simulink model "UWV_SIM"  (R2017a)
settings: Solver=FixedStepAuto  StartTime=0.0  StopTime=5  FixedStep=0.01  RelTol=1e-3  EnableMultiTasking=on
settings Model: Creator=Think  LastModifiedBy=Think
settings DataIOCC: LimitDataPoints=on  SaveFormat=Array
settings OptimizationCC: LifeSpan=inf
settings DebuggingCC: SolverPrmCheckMsg=warning  SFUnexpectedBacktrackingDiag=warning  SFNoUnconditionalDefaultTransitionDiag=warning  SFExecutionAtInitializationDiag=none
settings HardwareCC: ProdBitPerPointer=32  ProdBitPerSizeT=32  ProdBitPerPtrDiffT=32  ProdLargestAtomicFloat=None  ProdIntDivRoundTo=Undefined  ProdEndianess=Unspecified  ProdWordSize=32  ProdHWDeviceType=32-bit Generic
settings ModelReferenceCC: PropagateSignalLabelsOutOfModel=off
settings GRTTargetCC: TargetLangStandard=C89/C90 (ANSI)  GeneratePreprocessorConditionals=Disable all
settings ConfigComp: CovMetricSettings=dw  CovHtmlReporting=on  CovSaveCumulativeToWorkspaceVar=on  CovSaveSingleToWorkspaceVar=on  CovExternalEMLEnable=off  CovSFcnEnable=off

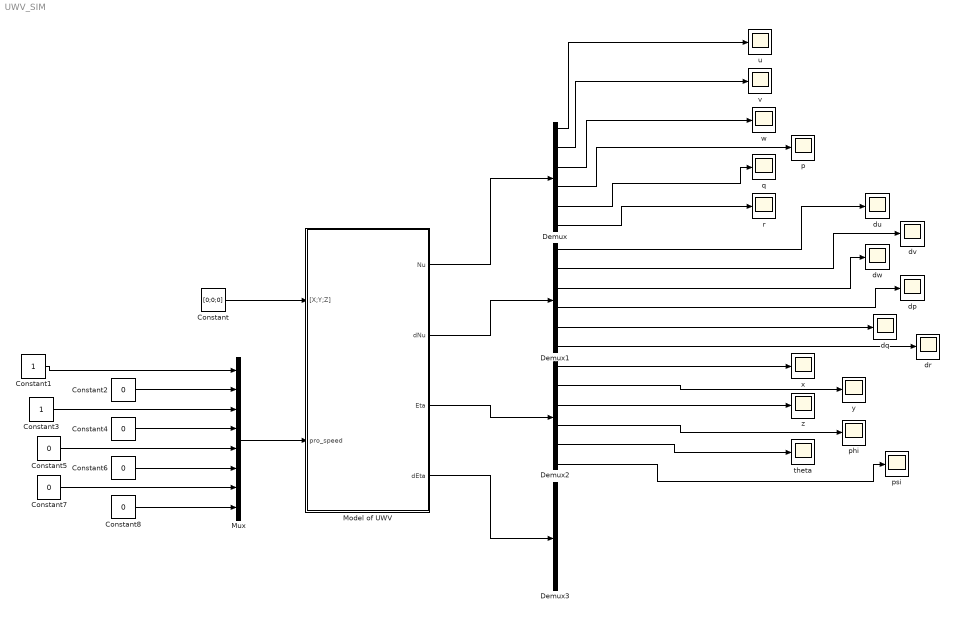
== system UWV_SIM ==
  Constant : Constant  Value=[0;0;0]
  Constant1 : Constant
  Constant{2,4..8} (6 alike) : Constant  Value=0
  Constant3 : Constant
  Demux{,1..3} (4 alike) : Demux  Outputs=6
  Model of UWV : Subsystem
  Mux : Mux  Inputs=8
  dp : Scope
  dq : Scope
  dr : Scope
  du : Scope
  dv : Scope
  dw : Scope
  p : Scope
  phi : Scope
  psi : Scope
  q : Scope
  r : Scope
  theta : Scope
  u : Scope
  v : Scope
  w : Scope
  x : Scope
  y : Scope
  z : Scope
  wires:
  Constant/1 -> Model of UWV/1("[X;Y;Z]")
  Mux/1 -> Model of UWV/2(pro_speed)
  Model of UWV/1(Nu) -> Demux/1
  Model of UWV/2(dNu) -> Demux1/1
  Model of UWV/3(Eta) -> Demux2/1
  Model of UWV/4(dEta) -> Demux3/1
  Demux/1 -> u/1
  Demux/2 -> v/1
  Demux/3 -> w/1
  Demux/4 -> p/1
  Demux/5 -> q/1
  Demux/6 -> r/1
  Demux1/1 -> du/1
  Demux1/2 -> dv/1
  Demux1/3 -> dw/1
  Demux1/4 -> dp/1
  Demux1/5 -> dq/1
  Demux1/6 -> dr/1
  Demux2/1 -> x/1
  Demux2/2 -> y/1
  Demux2/3 -> z/1
  Demux2/4 -> phi/1
  Demux2/5 -> theta/1
  Demux2/6 -> psi/1
  Constant1/1 -> Mux/1
  Constant3/1 -> Mux/3
  Constant5/1 -> Mux/5
  Constant7/1 -> Mux/7
  Constant2/1 -> Mux/2
  Constant4/1 -> Mux/4
  Constant6/1 -> Mux/6
  Constant8/1 -> Mux/8

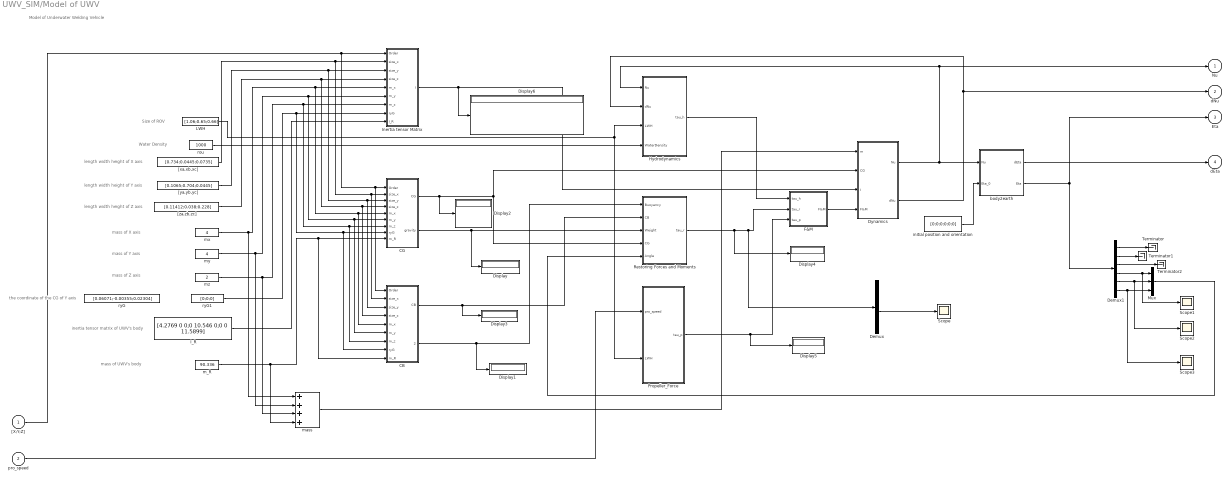
== system UWV_SIM/Model of UWV ==
  note: length width height of X axis
  note: Model of Underwater Welding Vehicle
  note: length width height of Y axis
  note: length width height of Z axis
  note: mass of X axis
  note: mass of Y axis
  note: mass of Z axis
  note: the coordinate of the CG of Y axis
  note: inertia tensor matrix of UWV's body
  note: mass of UWV's body
  note: Water Density
  note: Size of ROV
  "[X;Y;Z]" : Inport
  pro_speed : Inport  Port=2
  CB : Subsystem
  CG : Subsystem
  Demux : Demux  Outputs=6
  Demux1 : Demux  Outputs=6
  Display{,1..6} (7 alike) : Display
  Dynamics : Subsystem
  F&M : Subsystem
  Hydrodynamics : Subsystem
  I_R : Constant  Value=[4.2769 0 0;0 10.546 0;0 0 11.5899]
  Inertia tensor Matrix : Subsystem
  LWH : Constant  Value=[1.06;0.65;0.66]
  Mux : Mux  Inputs=3
  Propeller_Force : Subsystem
  Restoring Forces and Moments : Subsystem
  Scope{,1..3} (4 alike) : Scope
  Terminator : Terminator
  Terminator1 : Terminator
  Terminator2 : Terminator
  "[xa,xb,xc]" : Constant  Value=[0.734;0.0445;0.0735]
  "[ya,yb,yc]" : Constant  Value=[0.1065;0.704;0.0445]
  "[za,zb,zc]" : Constant  Value=[0.11412;0.038;0.228]
  "body2earth " : Subsystem
  initial position and orientation : Constant  Value=[0;0;0;0;0;0]
  m_R : Constant  Value=90.336
  mass : Sum  Inputs=++++
      mask Display:
      | port_label('input',1,'m_x')
      | port_label('input',2,'m_y')
      | port_label('input',3,'m_z')
      | port_label('input',4,'m_R')
      | port_label('output',1,'m')
  mx : Constant  Value=4
  my : Constant  Value=4
  mz : Constant  Value=2
  rou : Constant  Value=1000
  ryG : Constant  Value=[0.06071;-0.00355;0.02304]
  ryG1 : Constant  Value=[0;0;0]
  Nu : Outport
  dNu : Outport  Port=2
  Eta : Outport  Port=3
  dEta : Outport  Port=4
  wires:
  "body2earth "/2(Eta) -> Demux1/1, Eta/1
  "body2earth "/1(dEta) -> dEta/1
  initial position and orientation/1 -> "body2earth "/2(Eta_0)
  "[X;Y;Z]"/1 -> Inertia tensor Matrix/1(Order), CB/1(Order), CG/1(Order)
  "[xa,xb,xc]"/1 -> CB/2(size_x), CG/2(size_x), Inertia tensor Matrix/2(size_x)
  "[ya,yb,yc]"/1 -> CB/3(size_y), CG/3(size_y), Inertia tensor Matrix/3(size_y)
  "[za,zb,zc]"/1 -> CB/4(size_z), CG/4(size_z), Inertia tensor Matrix/4(size_z)
  mx/1 -> mass/1, CB/5(m_x), CG/5(m_x), Inertia tensor Matrix/5(m_x)
  my/1 -> mass/2, CB/6(m_y), CG/6(m_y), Inertia tensor Matrix/6(m_y)
  mz/1 -> mass/3, CB/7(m_z), CG/7(m_z), Inertia tensor Matrix/7(m_z)
  ryG1/1 -> CB/8(ryG), CG/8(ryG), Inertia tensor Matrix/8(ryG)
  I_R/1 -> Inertia tensor Matrix/9(I_R)
  m_R/1 -> mass/4, CB/9(m_R), CG/9(m_R)
  CB/1(CB) -> Display3/1, Restoring Forces and Moments/2(CB)
  CG/2(gravity) -> Display/1, Restoring Forces and Moments/3(Weight)
  CB/2(Buoyancy) -> Display1/1, Restoring Forces and Moments/1(Buoyancy)
  Dynamics/1(Nu) -> "body2earth "/1(Nu), Hydrodynamics/1(Nu), Nu/1
  Demux1/4 -> Scope1/1, Mux/1
  Demux1/5 -> Scope2/1, Mux/2
  Demux1/6 -> Scope3/1, Mux/3
  CG/1(CG) -> Display2/1, Restoring Forces and Moments/4(CG), Dynamics/2(CG)
  mass/1 -> Dynamics/1(m)
  Dynamics/2(dNu) -> Hydrodynamics/2(dNu), dNu/1
  Mux/1 -> Restoring Forces and Moments/5(Angle)
  F&M/1(F&M) -> Dynamics/4(F&M)
  Restoring Forces and Moments/1(tau_r) -> Display4/1, Demux/1, F&M/2(tau_r)
  Inertia tensor Matrix/1(I) -> Display6/1, Dynamics/3(I)
  rou/1 -> Hydrodynamics/4(WaterDensity)
  LWH/1 -> Propeller_Force/2(LWH), Hydrodynamics/3(LWH)
  pro_speed/1 -> Propeller_Force/1(pro_speed)
  Propeller_Force/1(tau_p) -> Display5/1, F&M/3(tau_p)
  Demux1/1 -> Terminator/1
  Demux1/2 -> Terminator1/1
  Demux1/3 -> Terminator2/1
  Demux/4 -> Scope/1
  Hydrodynamics/1(tau_h) -> F&M/1(tau_h)

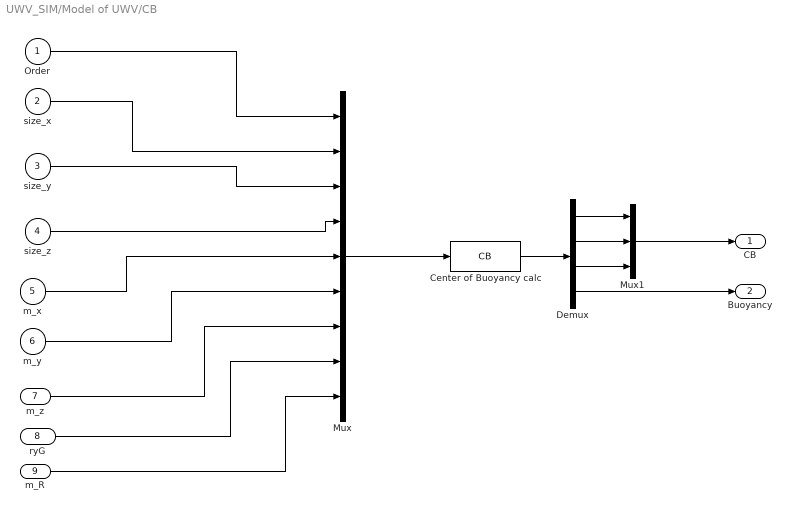
== system UWV_SIM/Model of UWV/CB ==
  Order : Inport
  size_x : Inport  Port=2
  size_y : Inport  Port=3
  size_z : Inport  Port=4
  m_x : Inport  Port=5
  m_y : Inport  Port=6
  m_z : Inport  Port=7
  ryG : Inport  Port=8
  m_R : Inport  Port=9
  Center of Buoyancy calc : MATLABFcn  MATLABFcn=CB  Output1D=off
  Demux : Demux
  Mux : Mux  Inputs=9
  Mux1 : Mux  Inputs=3
  CB : Outport
  Buoyancy : Outport  Port=2
  wires:
  m_x/1 -> Mux/5
  m_y/1 -> Mux/6
  size_x/1 -> Mux/2
  ryG/1 -> Mux/8
  size_z/1 -> Mux/4
  Order/1 -> Mux/1
  size_y/1 -> Mux/3
  m_R/1 -> Mux/9
  m_z/1 -> Mux/7
  Mux/1 -> Center of Buoyancy calc/1
  Center of Buoyancy calc/1 -> Demux/1
  Demux/1 -> Mux1/1
  Demux/2 -> Mux1/2
  Demux/3 -> Mux1/3
  Demux/4 -> Buoyancy/1
  Mux1/1 -> CB/1

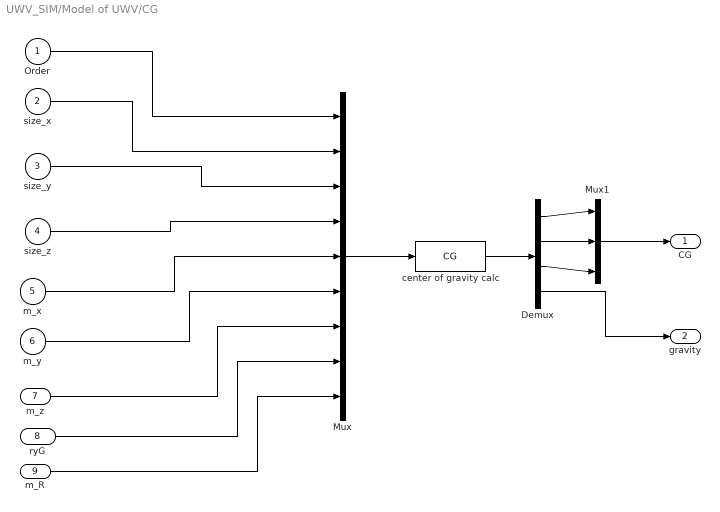
== system UWV_SIM/Model of UWV/CG ==
  Order : Inport
  size_x : Inport  Port=2
  size_y : Inport  Port=3
  size_z : Inport  Port=4
  m_x : Inport  Port=5
  m_y : Inport  Port=6
  m_z : Inport  Port=7
  ryG : Inport  Port=8
  m_R : Inport  Port=9
  Demux : Demux
  Mux : Mux  Inputs=9
  Mux1 : Mux  Inputs=3
  center of gravity calc : MATLABFcn  MATLABFcn=CG  Output1D=off
  CG : Outport
  gravity : Outport  Port=2
  wires:
  m_R/1 -> Mux/9
  Mux/1 -> center of gravity calc/1
  ryG/1 -> Mux/8
  Order/1 -> Mux/1
  m_z/1 -> Mux/7
  size_y/1 -> Mux/3
  size_z/1 -> Mux/4
  m_x/1 -> Mux/5
  size_x/1 -> Mux/2
  m_y/1 -> Mux/6
  center of gravity calc/1 -> Demux/1
  Demux/1 -> Mux1/1
  Demux/2 -> Mux1/2
  Demux/3 -> Mux1/3
  Mux1/1 -> CG/1
  Demux/4 -> gravity/1

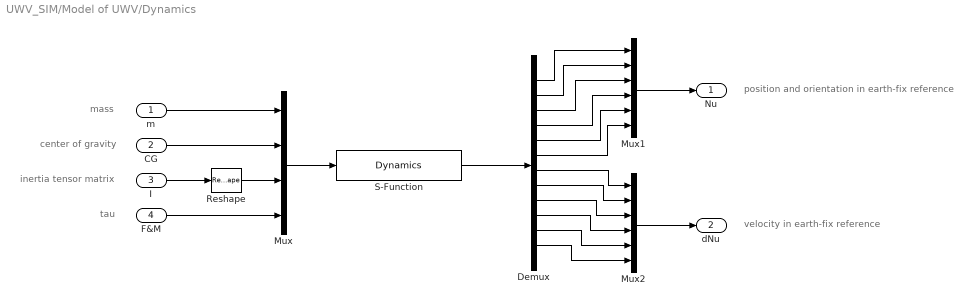
== system UWV_SIM/Model of UWV/Dynamics ==
  note: velocity in earth-fix reference
  note: inertia tensor matrix
  note: tau
  note: center of gravity
  note: mass
  note: position and orientation in earth-fix reference
  m : Inport
  CG : Inport  Port=2
  I : Inport  Port=3
  F&M : Inport  Port=4
  Demux : Demux  Outputs=12
  Mux : Mux
  Mux1 : Mux  Inputs=6
  Mux2 : Mux  Inputs=6
  Reshape : Reshape
  S-Function : S-Function  FunctionName=Dynamics  SFunctionDeploymentMode=off  EnableBusSupport=off
  Nu : Outport
  dNu : Outport  Port=2
  wires:
  CG/1 -> Mux/2
  I/1 -> Reshape/1
  m/1 -> Mux/1
  Reshape/1 -> Mux/3
  F&M/1 -> Mux/4
  Mux/1 -> S-Function/1
  S-Function/1 -> Demux/1
  Demux/1 -> Mux1/1
  Demux/2 -> Mux1/2
  Demux/3 -> Mux1/3
  Demux/4 -> Mux1/4
  Demux/5 -> Mux1/5
  Demux/6 -> Mux1/6
  Mux1/1 -> Nu/1
  Demux/7 -> Mux2/1
  Demux/8 -> Mux2/2
  Demux/9 -> Mux2/3
  Demux/10 -> Mux2/4
  Demux/11 -> Mux2/5
  Demux/12 -> Mux2/6
  Mux2/1 -> dNu/1

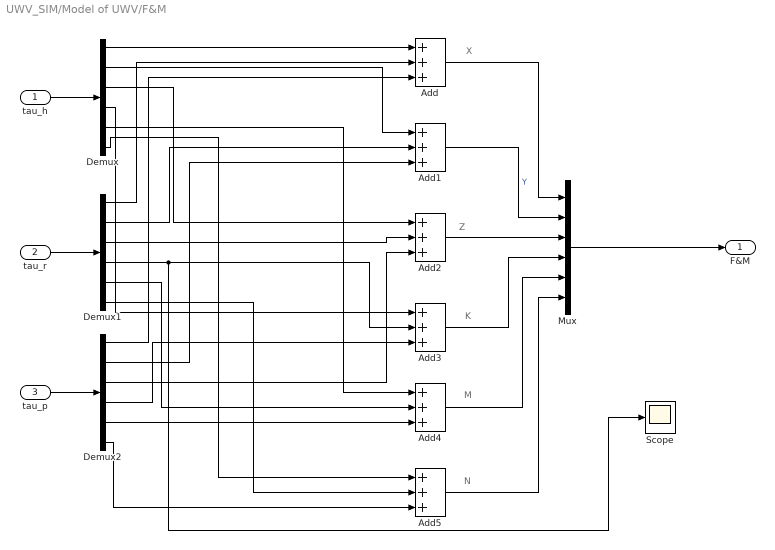
== system UWV_SIM/Model of UWV/F&M ==
  note: N
  note: M
  note: K
  note: Z
  note: X
  tau_h : Inport
  tau_r : Inport  Port=2
  tau_p : Inport  Port=3
  Add{,1..5} (6 alike) : Sum  Inputs=+++
  Demux : Demux  Outputs=6
  Demux1 : Demux  Outputs=6
  Demux2 : Demux  Outputs=6
  Mux : Mux  Inputs=6
  Scope : Scope
  F&M : Outport
  wires:
  tau_h/1 -> Demux/1
  tau_r/1 -> Demux1/1
  tau_p/1 -> Demux2/1
  Demux/1 -> Add/1
  Demux1/1 -> Add/2
  Demux2/1 -> Add/3
  Demux/2 -> Add1/1
  Demux1/2 -> Add1/2
  Demux2/2 -> Add1/3
  Demux/3 -> Add2/1
  Demux1/3 -> Add2/2
  Demux2/3 -> Add2/3
  Demux/4 -> Add3/1
  Demux1/4 -> Scope/1, Add3/2
  Demux2/4 -> Add3/3
  Demux/5 -> Add4/1
  Demux1/5 -> Add4/2
  Demux2/5 -> Add4/3
  Demux/6 -> Add5/1
  Demux1/6 -> Add5/2
  Demux2/6 -> Add5/3
  Add/1 -> Mux/1
  Add1/1 -> Mux/2  "Y"
  Add2/1 -> Mux/3
  Add3/1 -> Mux/4
  Add4/1 -> Mux/5
  Add5/1 -> Mux/6
  Mux/1 -> F&M/1

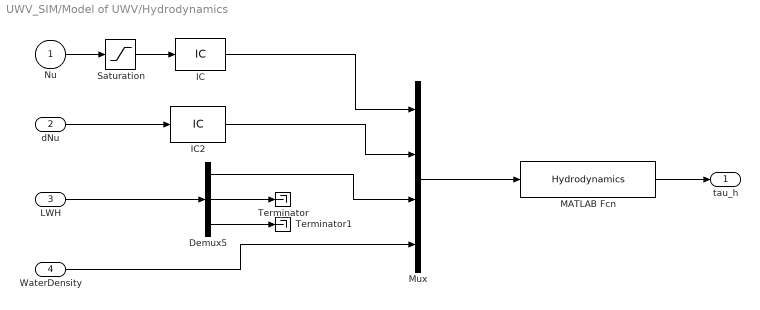
== system UWV_SIM/Model of UWV/Hydrodynamics ==
  Nu : Inport
  dNu : Inport  Port=2
  LWH : Inport  Port=3
  WaterDensity : Inport  Port=4
  Demux5 : Demux  Outputs=3
  IC : InitialCondition  Value=0.001
  IC2 : InitialCondition  Value=0.001
  MATLAB Fcn : MATLABFcn  MATLABFcn=Hydrodynamics  OutputDimensions=6  Output1D=off
  Mux : Mux
  Saturation : Saturate  UpperLimit=0.8  LowerLimit=-0.8
  Terminator : Terminator
  Terminator1 : Terminator
  tau_h : Outport
  wires:
  MATLAB Fcn/1 -> tau_h/1
  Mux/1 -> MATLAB Fcn/1
  LWH/1 -> Demux5/1
  Demux5/2 -> Terminator/1
  Demux5/3 -> Terminator1/1
  Nu/1 -> Saturation/1
  dNu/1 -> IC2/1
  Saturation/1 -> IC/1
  IC/1 -> Mux/1
  IC2/1 -> Mux/2
  Demux5/1 -> Mux/3
  WaterDensity/1 -> Mux/4

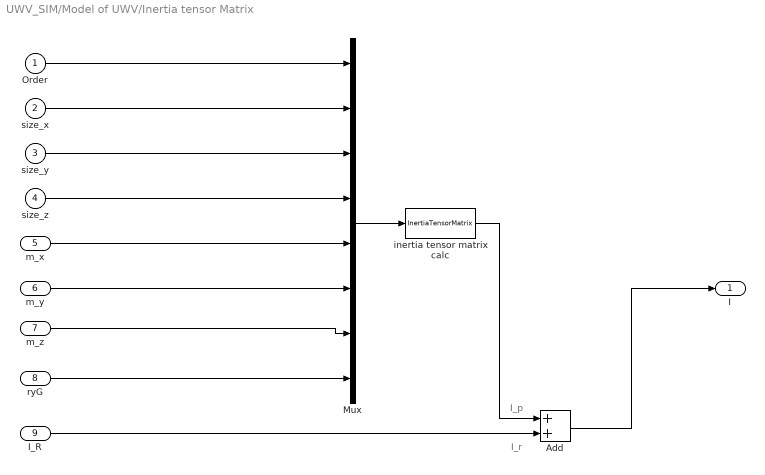
== system UWV_SIM/Model of UWV/Inertia tensor Matrix ==
  note: I_r
  note: I_p
  Order : Inport
  size_x : Inport  Port=2
  size_y : Inport  Port=3
  size_z : Inport  Port=4
  m_x : Inport  Port=5
  m_y : Inport  Port=6
  m_z : Inport  Port=7
  ryG : Inport  Port=8
  I_R : Inport  Port=9
  Add : Sum
  Mux : Mux  Inputs=8
  inertia tensor matrix calc : MATLABFcn  MATLABFcn=InertiaTensorMatrix  Output1D=off
  I : Outport
  wires:
  inertia tensor matrix calc/1 -> Add/1
  I_R/1 -> Add/2
  Mux/1 -> inertia tensor matrix calc/1
  m_z/1 -> Mux/7
  size_z/1 -> Mux/4
  m_x/1 -> Mux/5
  Order/1 -> Mux/1
  m_y/1 -> Mux/6
  size_x/1 -> Mux/2
  size_y/1 -> Mux/3
  ryG/1 -> Mux/8
  Add/1 -> I/1

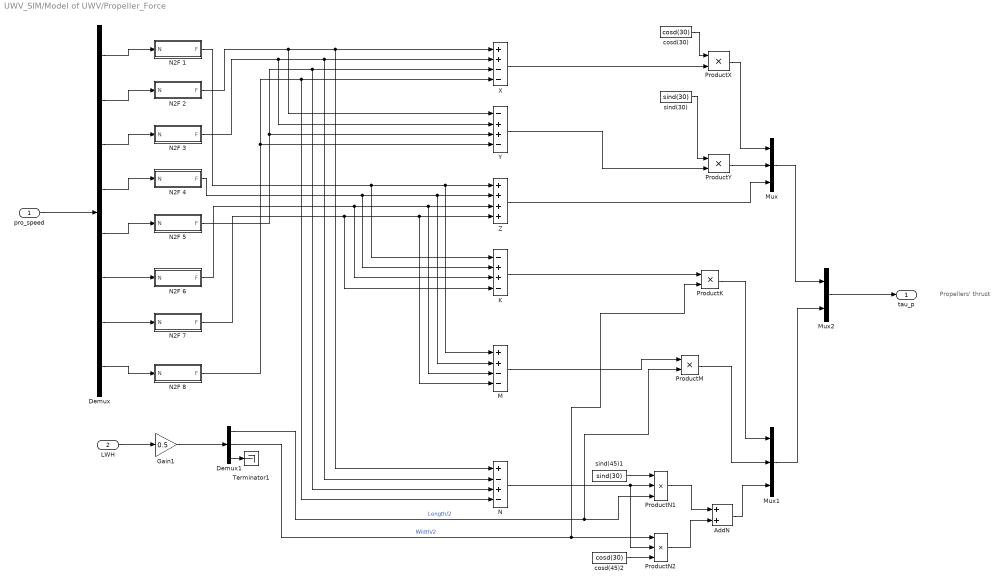
== system UWV_SIM/Model of UWV/Propeller_Force ==
  note: Propellers' thrust
  pro_speed : Inport
  LWH : Inport  Port=2
  AddN : Sum
  Demux : Demux  Outputs=8
  Demux1 : Demux  Outputs=3
  Gain1 : Gain  Gain=0.5
  K : Sum  Inputs=-++-
  M : Sum  Inputs=++--
  Mux : Mux  Inputs=3
  Mux1 : Mux  Inputs=3
  Mux2 : Mux  Inputs=2
  N : Sum  Inputs=+-+-
  N2F 1 : Subsystem
  N2F 2 : Subsystem
  N2F 3 : Subsystem
  N2F 4 : Subsystem
  N2F 5 : Subsystem
  N2F 6 : Subsystem
  N2F 7 : Subsystem
  N2F 8 : Subsystem
  ProductK : Product
  ProductM : Product
  ProductN1 : Product  Inputs=3
  ProductN2 : Product  Inputs=3
  ProductX : Product
  ProductY : Product
  Terminator1 : Terminator
  X : Sum  Inputs=++--
  Y : Sum  Inputs=-++-
  Z : Sum  Inputs=++++
  cosd(30) : Constant  Value=cosd(30)
  cosd(45)2 : Constant  Value=cosd(30)
  sind(30) : Constant  Value=sind(30)
  sind(45)1 : Constant  Value=sind(30)
  tau_p : Outport
  wires:
  Mux1/1 -> Mux2/2
  Mux/1 -> Mux2/1
  X/1 -> ProductX/2
  ProductX/1 -> Mux/1
  ProductY/1 -> Mux/2
  Y/1 -> ProductY/2
  Z/1 -> Mux/3
  Demux1/3 -> Terminator1/1
  Gain1/1 -> Demux1/1
  LWH/1 -> Gain1/1
  cosd(30)/1 -> ProductX/1
  sind(30)/1 -> ProductY/1
  N/1 -> ProductN2/2, ProductN1/2
  sind(45)1/1 -> ProductN1/1
  cosd(45)2/1 -> ProductN2/3
  Demux1/1 -> ProductM/2, ProductN1/3  "Length/2"
  Demux1/2 -> ProductN2/1, ProductK/2  "Width/2"
  ProductN1/1 -> AddN/1
  ProductN2/1 -> AddN/2
  AddN/1 -> Mux1/3
  K/1 -> ProductK/1
  M/1 -> ProductM/1
  ProductK/1 -> Mux1/1
  ProductM/1 -> Mux1/2
  Mux2/1 -> tau_p/1
  N2F 2/1(F) -> Y/1, X/1, N/1
  N2F 3/1(F) -> Y/2, X/2, N/2
  N2F 5/1(F) -> X/3, N/3, Y/3
  N2F 8/1(F) -> X/4, N/4, Y/4
  N2F 4/1(F) -> K/2, M/2, Z/2
  N2F 6/1(F) -> K/3, M/3, Z/3
  N2F 1/1(F) -> K/1, M/1, Z/1
  N2F 7/1(F) -> K/4, M/4, Z/4
  Demux/8 -> N2F 8/1(N)
  Demux/1 -> N2F 1/1(N)
  Demux/2 -> N2F 2/1(N)
  Demux/3 -> N2F 3/1(N)
  Demux/4 -> N2F 4/1(N)
  Demux/5 -> N2F 5/1(N)
  Demux/6 -> N2F 6/1(N)
  Demux/7 -> N2F 7/1(N)
  pro_speed/1 -> Demux/1

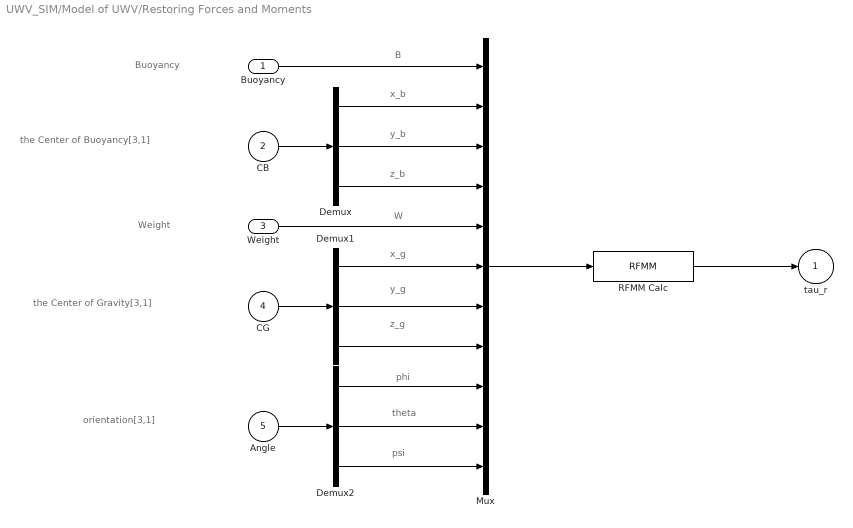
== system UWV_SIM/Model of UWV/Restoring Forces and Moments ==
  note: psi
  note: theta
  note: phi
  note: W
  note: x_b
  note: B
  note: Buoyancy
  note: the Center of Buoyancy[3,1]
  note: Weight
  note: the Center of Gravity[3,1]
  note: orientation[3,1]
  note: y_b
  note: z_b
  note: x_g
  note: y_g
  note: z_g
  Buoyancy : Inport
  CB : Inport  Port=2
  Weight : Inport  Port=3
  CG : Inport  Port=4
  Angle : Inport  Port=5
  Demux : Demux  Outputs=3
  Demux1 : Demux  Outputs=3
  Demux2 : Demux  Outputs=3
  Mux : Mux  Inputs=11
  RFMM Calc : MATLABFcn  MATLABFcn=RFMM  OutputDimensions=6
  tau_r : Outport
  wires:
  CB/1 -> Demux/1
  CG/1 -> Demux1/1
  Angle/1 -> Demux2/1
  Buoyancy/1 -> Mux/1
  Demux/1 -> Mux/2
  Demux/2 -> Mux/3
  Demux/3 -> Mux/4
  Weight/1 -> Mux/5
  Demux1/1 -> Mux/6
  Demux1/2 -> Mux/7
  Demux1/3 -> Mux/8
  Demux2/1 -> Mux/9
  Demux2/2 -> Mux/10
  Demux2/3 -> Mux/11
  Mux/1 -> RFMM Calc/1
  RFMM Calc/1 -> tau_r/1

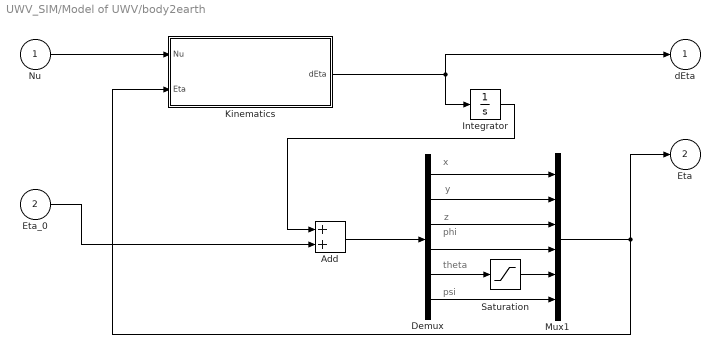
== system UWV_SIM/Model of UWV/body2earth  ==
  note: psi
  note: theta
  note: phi
  note: z
  note: y
  note: x
  Nu : Inport
  Eta_0 : Inport  Port=2
  Add : Sum
  Demux : Demux  Outputs=6
  Integrator : Integrator
  Kinematics : Subsystem
  Mux1 : Mux  Inputs=6
  Saturation : Saturate  UpperLimit=1.4  LowerLimit=-1.4
  dEta : Outport
  Eta : Outport  Port=2
  wires:
  Integrator/1 -> Add/1
  Eta_0/1 -> Add/2
  Add/1 -> Demux/1
  Demux/1 -> Mux1/1
  Demux/2 -> Mux1/2
  Demux/3 -> Mux1/3
  Demux/4 -> Mux1/4
  Demux/6 -> Mux1/6
  Demux/5 -> Saturation/1
  Saturation/1 -> Mux1/5
  Mux1/1 -> Kinematics/2(Eta), Eta/1
  Kinematics/1(dEta) -> dEta/1, Integrator/1
  Nu/1 -> Kinematics/1(Nu)

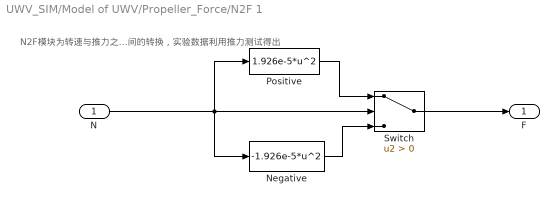
== system UWV_SIM/Model of UWV/Propeller_Force/N2F 1 ==
  note: N2F模块为转速与推力之间的转换，实验数据利用推力测试得出
  N : Inport
  Negative : Fcn  Expr=-1.926e-5*u^2
  Positive : Fcn  Expr=1.926e-5*u^2
  Switch : Switch  Criteria=u2 > Threshold
  F : Outport
  wires:
  N/1 -> Negative/1, Positive/1, Switch/2
  Switch/1 -> F/1
  Positive/1 -> Switch/1
  Negative/1 -> Switch/3

== system UWV_SIM/Model of UWV/Propeller_Force/N2F 2 ==
  note: N2F模块为转速与推力之间的转换，实验数据利用推力测试得出
  N : Inport
  Negative : Fcn  Expr=-1.926e-5*u^2
  Positive : Fcn  Expr=1.926e-5*u^2
  Switch : Switch  Criteria=u2 > Threshold
  F : Outport
  wires:
  N/1 -> Negative/1, Positive/1, Switch/2
  Switch/1 -> F/1
  Positive/1 -> Switch/1
  Negative/1 -> Switch/3

== system UWV_SIM/Model of UWV/Propeller_Force/N2F 3 ==
  note: N2F模块为转速与推力之间的转换，实验数据利用推力测试得出
  N : Inport
  Negative : Fcn  Expr=-1.926e-5*u^2
  Positive : Fcn  Expr=1.926e-5*u^2
  Switch : Switch  Criteria=u2 > Threshold
  F : Outport
  wires:
  N/1 -> Negative/1, Positive/1, Switch/2
  Switch/1 -> F/1
  Positive/1 -> Switch/1
  Negative/1 -> Switch/3

== system UWV_SIM/Model of UWV/Propeller_Force/N2F 4 ==
  note: N2F模块为转速与推力之间的转换，实验数据利用推力测试得出
  N : Inport
  Negative : Fcn  Expr=-1.926e-5*u^2
  Positive : Fcn  Expr=1.926e-5*u^2
  Switch : Switch  Criteria=u2 > Threshold
  F : Outport
  wires:
  N/1 -> Negative/1, Positive/1, Switch/2
  Switch/1 -> F/1
  Positive/1 -> Switch/1
  Negative/1 -> Switch/3

== system UWV_SIM/Model of UWV/Propeller_Force/N2F 5 ==
  note: N2F模块为转速与推力之间的转换，实验数据利用推力测试得出
  N : Inport
  Negative : Fcn  Expr=-1.926e-5*u^2
  Positive : Fcn  Expr=1.926e-5*u^2
  Switch : Switch  Criteria=u2 > Threshold
  F : Outport
  wires:
  N/1 -> Negative/1, Positive/1, Switch/2
  Switch/1 -> F/1
  Positive/1 -> Switch/1
  Negative/1 -> Switch/3

== system UWV_SIM/Model of UWV/Propeller_Force/N2F 6 ==
  note: N2F模块为转速与推力之间的转换，实验数据利用推力测试得出
  N : Inport
  Negative : Fcn  Expr=-1.926e-5*u^2
  Positive : Fcn  Expr=1.926e-5*u^2
  Switch : Switch  Criteria=u2 > Threshold
  F : Outport
  wires:
  N/1 -> Negative/1, Positive/1, Switch/2
  Switch/1 -> F/1
  Positive/1 -> Switch/1
  Negative/1 -> Switch/3

== system UWV_SIM/Model of UWV/Propeller_Force/N2F 7 ==
  note: N2F模块为转速与推力之间的转换，实验数据利用推力测试得出
  N : Inport
  Negative : Fcn  Expr=-1.926e-5*u^2
  Positive : Fcn  Expr=1.926e-5*u^2
  Switch : Switch  Criteria=u2 > Threshold
  F : Outport
  wires:
  N/1 -> Negative/1, Positive/1, Switch/2
  Switch/1 -> F/1
  Positive/1 -> Switch/1
  Negative/1 -> Switch/3

== system UWV_SIM/Model of UWV/Propeller_Force/N2F 8 ==
  note: N2F模块为转速与推力之间的转换，实验数据利用推力测试得出
  N : Inport
  Negative : Fcn  Expr=-1.926e-5*u^2
  Positive : Fcn  Expr=1.926e-5*u^2
  Switch : Switch  Criteria=u2 > Threshold
  F : Outport
  wires:
  N/1 -> Negative/1, Positive/1, Switch/2
  Switch/1 -> F/1
  Positive/1 -> Switch/1
  Negative/1 -> Switch/3

== system UWV_SIM/Model of UWV/body2earth /Kinematics ==
  Nu : Inport
  Eta : Inport  Port=2
  Kinematics Calc : MATLABFcn  MATLABFcn=Kinematics
  Mux : Mux  Inputs=2
  dEta : Outport
  wires:
  Kinematics Calc/1 -> dEta/1
  Nu/1 -> Mux/1
  Mux/1 -> Kinematics Calc/1
  Eta/1 -> Mux/2
